simulink model "TamiyaRobotExample_V15"  (R2024b)
settings: Solver=FixedStepAuto  StartTime=0.0  StopTime=inf  FixedStep=1/10  RelTol=1e-3
libraries: mbedblockslib x8
settings Model: ExtModeTrigDuration=5  Creator=The MathWorks, Inc.  LastModifiedBy=totani
settings SolverCC: AlgebraicLoopSolver=TrustRegion
settings DataIOCC: LimitDataPoints=on  ReturnWorkspaceOutputs=off
settings OptimizationCC: BlockReduction=off  LifeSpan=Inf  MaxStackSize=64
settings DebuggingCC: UnconnectedInputMsg=warning  UnconnectedOutputMsg=warning  UnconnectedLineMsg=warning  AllowSymbolicDim=off  SFUnexpectedBacktrackingDiag=warning  SFNoUnconditionalDefaultTransitionDiag=warning  SFExecutionAtInitializationDiag=none  ArithmeticOperatorsInVariantConditions=warning
settings HardwareCC: ProdBitPerPointer=32  ProdBitPerSizeT=32  ProdBitPerPtrDiffT=32  ProdLargestAtomicInteger=Long  ProdLargestAtomicFloat=Double  ProdWordSize=32  ProdHWDeviceType=ARM Compatible->ARM Cortex
settings ModelReferenceCC: EnableRefExpFcnMdlSchedulingChecks=on  PropagateSignalLabelsOutOfModel=off
settings SFSimCC: SimUseLocalCustomCode=off  CustomCodeUndefinedFunction=UseInterfaceOnly
settings RTWCC: Description=Embedded Coder  SystemTargetFile=ert.tlc  HardwareBoard=BBC micro:bit V1.5  TemplateMakefile=ert_default_tmf  RTWUseLocalCustomCode=off  Toolchain=GNU Tools for ARM Embedded Processors  BuildConfiguration=Faster Runs  GPUComputeCapability=3.5
settings CodeAppCC: StateflowObjectComments=on
settings ERTTargetCC: MultiwordLength=2048  ERTCustomFileBanners=off  SupportContinuousTime=on  SupportNonInlinedSFcns=on  RemoveResetFunc=off  ModelStepFunctionPrototypeControlCompliant=off  ExtModeTransport=3  ExtModeStaticAlloc=on  ExtModeMexFile=ext_xcp  ExtModeIntrfLevel=Level2 - Open  InlinedParameterPlacement=Hierarchical  ConvertIfToSwitch=off  SuppressUnreachableDefaultCases=off  DynamicArrayContainerType=coder::array
settings ConfigComp: CovMetricSettings=dw  CovSaveCumulativeToWorkspaceVar=on  CovSaveSingleToWorkspaceVar=on  CovExternalEMLEnable=off

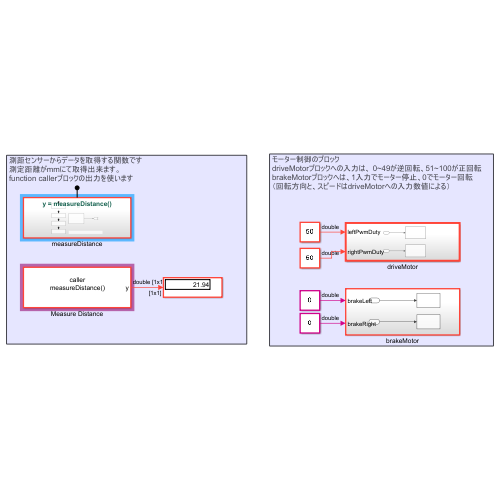
[thumbnail: Simulink's stored preview of the top-level diagram]
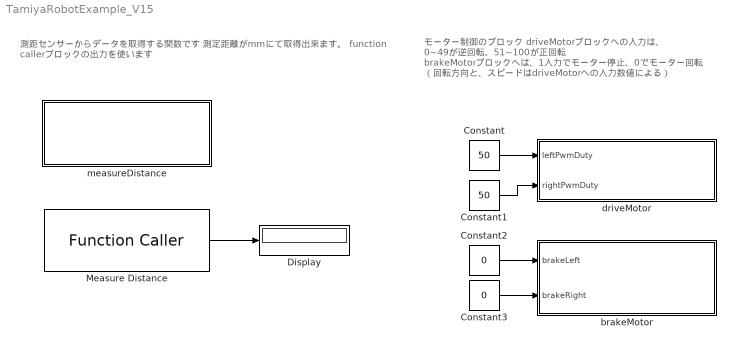
== system TamiyaRobotExample_V15 ==
  note: モーター制御のブロック
      | driveMotorブロックへの入力は、 0~49が逆回転、51~100が正回転
      | brakeMotorブロックへは、1入力でモーター停止、0でモーター回転
      | （回転方向と、スピードはdriveMotorへの入力数値による）
  note: 測距センサーからデータを取得する関数です
      | 測定距離がmmにて取得出来ます。
      | function callerブロックの出力を使います
  Constant : Constant  Value=50  SampleTime=1/10
  Constant1 : Constant  Value=50  SampleTime=1/10
  Constant2 : Constant  Value=0
  Constant3 : Constant  Value=0
  Display : Display
  Measure Distance : FunctionCaller  FunctionPrototype=y = measureDistance()  InputArgumentSpecifications=<Enter example>  OutputArgumentSpecifications=double(1)  SampleTime=1/10
  brakeMotor : Subsystem
  driveMotor : Subsystem  TreatAsAtomicUnit=on
  measureDistance : Subsystem  TreatAsAtomicUnit=on
  wires:
  Constant/1 -> driveMotor/1(leftPwmDuty)
  Constant1/1 -> driveMotor/2(rightPwmDuty)
  Measure Distance/1 -> Display/1
  Constant2/1 -> brakeMotor/1(brakeLeft)
  Constant3/1 -> brakeMotor/2(brakeRight)

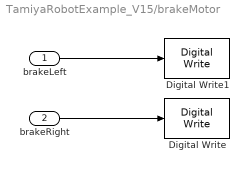
== system TamiyaRobotExample_V15/brakeMotor ==
  brakeLeft : Inport
  brakeRight : Inport  Port=2
  Digital Write : mbedblockslib/Digital Write  Pin=P15  Direction=output
  Digital Write1 : mbedblockslib/Digital Write  Pin=P16  Direction=output
  wires:
  brakeRight/1 -> Digital Write/1
  brakeLeft/1 -> Digital Write1/1

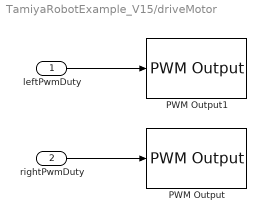
== system TamiyaRobotExample_V15/driveMotor ==
  leftPwmDuty : Inport
  rightPwmDuty : Inport  Port=2
  PWM Output : mbedblockslib/PWM Output  Pin=P13  EnableInputFrequency=off  InitialFrequency=1000  InitialDutyCycle=50  NotificationType=None
  PWM Output1 : mbedblockslib/PWM Output  Pin=P14  EnableInputFrequency=off  InitialFrequency=1000  InitialDutyCycle=50  NotificationType=None
  wires:
  leftPwmDuty/1 -> PWM Output1/1
  rightPwmDuty/1 -> PWM Output/1

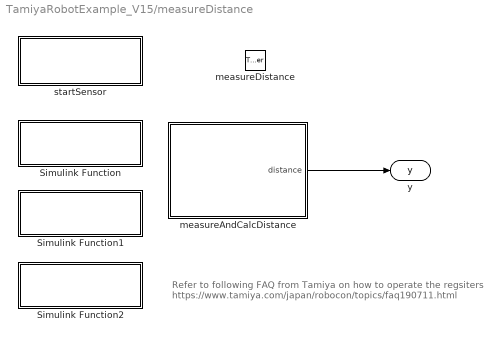
== system TamiyaRobotExample_V15/measureDistance ==
  note: Refer to following FAQ from Tamiya on how to operate the regsiters
      | https://www.tamiya.com/japan/robocon/topics/faq190711.html
  measureDistance : TriggerPort  TriggerType=function-call  IsSimulinkFunction=on  FunctionName=measureDistance  FunctionVisibility=scoped  VariantControl=(inherit)
  Simulink Function : Subsystem  TreatAsAtomicUnit=on
  Simulink Function1 : Subsystem  TreatAsAtomicUnit=on
  Simulink Function2 : Subsystem  TreatAsAtomicUnit=on
  measureAndCalcDistance : MATLAB Function  TreatAsAtomicUnit=on
  startSensor : Subsystem
  y : ArgOut  DisableCoverage=on  ArgumentName=y
  wires:
  measureAndCalcDistance/1(distance) -> y/1

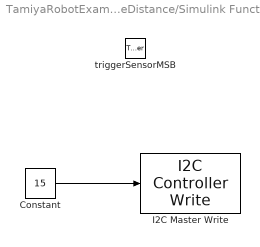
== system TamiyaRobotExample_V15/measureDistance/Simulink Function ==
  triggerSensorMSB : TriggerPort  TriggerType=function-call  IsSimulinkFunction=on  FunctionName=triggerSensorMSB  FunctionVisibility=scoped  VariantControl=(inherit)
  Constant : Constant  Value=15  OutDataTypeStr=uint8
  I2C Master Write : mbedblockslib/I2C Controller Write  I2CModule=0  Mode=Master  SlaveAddress=44  SlaveByteOrder=BigEndian  Direction=Transmitter  RegisterAddressMode=off  RegisterAddress=0  SlaveDataType=uint8  DataLength=1  NoAck=off  RepeatedStart=off  OutputStatus=off
  wires:
  Constant/1 -> I2C Master Write/1

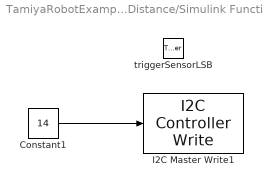
== system TamiyaRobotExample_V15/measureDistance/Simulink Function1 ==
  triggerSensorLSB : TriggerPort  TriggerType=function-call  IsSimulinkFunction=on  FunctionName=triggerSensorLSB  FunctionVisibility=scoped  VariantControl=(inherit)
  Constant1 : Constant  Value=14  OutDataTypeStr=uint8
  I2C Master Write1 : mbedblockslib/I2C Controller Write  I2CModule=0  Mode=Master  SlaveAddress=44  SlaveByteOrder=BigEndian  Direction=Transmitter  RegisterAddressMode=off  RegisterAddress=0  SlaveDataType=uint8  DataLength=1  NoAck=off  RepeatedStart=off  OutputStatus=off
  wires:
  Constant1/1 -> I2C Master Write1/1

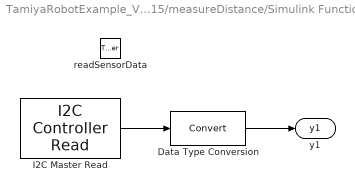
== system TamiyaRobotExample_V15/measureDistance/Simulink Function2 ==
  readSensorData : TriggerPort  TriggerType=function-call  IsSimulinkFunction=on  FunctionName=readSensorData  FunctionVisibility=scoped  VariantControl=(inherit)
  Data Type Conversion : DataTypeConversion  SaturateOnIntegerOverflow=off  RndMeth=Floor
  I2C Master Read : mbedblockslib/I2C Controller Read  I2CModule=0  Mode=Master  SlaveAddress=44  SlaveByteOrder=BigEndian  Direction=Receiver  RegisterAddressMode=off  RegisterAddress=0  SlaveDataType=uint8  DataLength=1  NoAck=off  RepeatedStart=off  OutputStatus=off  SampleTime=-1
  y1 : ArgOut  DisableCoverage=on  ArgumentName=y1
  wires:
  I2C Master Read/1 -> Data Type Conversion/1
  Data Type Conversion/1 -> y1/1

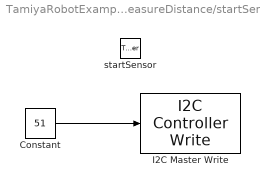
== system TamiyaRobotExample_V15/measureDistance/startSensor ==
  startSensor : TriggerPort  TriggerType=function-call  IsSimulinkFunction=on  FunctionName=startSensor  FunctionVisibility=scoped  VariantControl=(inherit)
  Constant : Constant  Value=51  OutDataTypeStr=uint8
  I2C Master Write : mbedblockslib/I2C Controller Write  I2CModule=0  Mode=Master  SlaveAddress=44  SlaveByteOrder=BigEndian  Direction=Transmitter  RegisterAddressMode=off  RegisterAddress=0  SlaveDataType=uint8  DataLength=1  NoAck=off  RepeatedStart=off  OutputStatus=off
  wires:
  Constant/1 -> I2C Master Write/1

== matlab function TamiyaRobotExample_V15/measureDistance/measureAndCalcDistance ==
  data: distance output
function distance = measureAndCalcDistance
%#codegen

startSensor();
readSensorData();

triggerSensorMSB();
msbData = readSensorData();
triggerSensorLSB();
lsbData = readSensorData();

%%
travelTime = (msbData*256+lsbData);
distance = (((travelTime - 160) / 2) * 0.315) / 10;
